simulink model "Vision"  (R2015a)
settings: Solver=ode45  SolverMode=SingleTasking  StartTime=0.0  StopTime=inf  RelTol=1e-3
undefined symbols (not defined in the file or in its folder): gray, none, strel, videoinput
libraries: simulink x12, visiontextngfix x6, visionanalysis x6, visionmorphops x4, visionstatistics x2, visionsinks x2, imaqlib x1
settings Model: CovMetricSettings=dwe  CovHtmlReporting=off  covSaveCumulativeToWorkspaceVar=off  CovSaveSingleToWorkspaceVar=off  CovExternalEMLEnable=on  Creator=Nauj_epilef  LastModifiedBy=Antonio
settings DataIOCC: LimitDataPoints=off  SaveFormat=Dataset
settings DebuggingCC: SFUnexpectedBacktrackingDiag=error  SFNoUnconditionalDefaultTransitionDiag=error
settings HardwareCC: ProdBitPerPointer=64  ProdLargestAtomicFloat=Float  ProdIntDivRoundTo=Zero  ProdEndianess=LittleEndian  ProdHWDeviceType=Specified
settings ModelReferenceCC: PropagateSignalLabelsOutOfModel=on
settings GRTTargetCC: TargetLangStandard=C99 (ISO)  GeneratePreprocessorConditionals=Use local settings

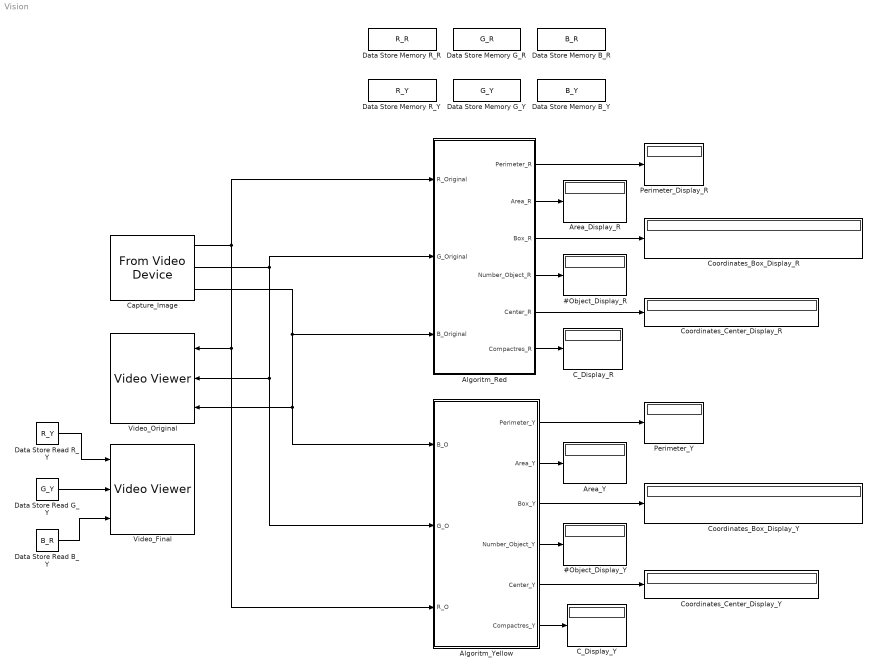
== system Vision ==
  #Object_Display_R : Display
  #Object_Display_Y : Display
  Algoritm_Red : Subsystem
  Algoritm_Yellow : Subsystem
  Area_Display_R : Display
  Area_Y : Display
  C_Display_R : Display
  "C_Display_Y " : Display
  Capture_Image : imaqlib/From Video Device  DeviceMenu=(none)  Device=winvideo 1 (Logitech HD Webcam C525)  ObjConstructor=videoinput('winvideo', 1)  VideoFormatMenu=(none)  VideoFormat=RGB24_640x480  VideoSource=input1  ROIPosition=[184 115 146 417]  EnableHWTrigger=off  TriggerConfiguration=none/none  SampleTime=1/10  OutputPortsMode=Separate color signals  DataType=single  CanDoHWTrigger=no  ReturnedColorSpace=rgb  BlockHandle=645.0004  ROIWidth=417  ROIHeight=146  ROIColumn=115  ROIRow=184  EngXMLPath=C:\Program Files\MATLAB\R2017a\toolbox\imaq\imaq\private  DevXMLPath=C:\ProgramData\MATLAB\SupportPackages\R2017a\toolbox\imaq\supportpackages\genericvideo\adaptor\win64  EngLibPath=C:\Program Files\MATLAB\R2017a\toolbox\imaq\imaqblks\imaqmex\win64  ColorSpace=rgb  BayerSensorAlignment=grbg
  Coordinates_Box_Display_R : Display
  Coordinates_Box_Display_Y : Display
  Coordinates_Center_Display_R : Display
  Coordinates_Center_Display_Y : Display
  Data Store Memory B_R : DataStoreMemory  DataStoreName=B_R  ReadBeforeWriteMsg=warning  WriteAfterWriteMsg=warning  WriteAfterReadMsg=warning  ShowAdditionalParam=off
  Data Store Memory B_Y : DataStoreMemory  DataStoreName=B_Y  ReadBeforeWriteMsg=warning  WriteAfterWriteMsg=warning  WriteAfterReadMsg=warning  ShowAdditionalParam=off
  Data Store Memory G_R : DataStoreMemory  DataStoreName=G_R  ReadBeforeWriteMsg=warning  WriteAfterWriteMsg=warning  WriteAfterReadMsg=warning  ShowAdditionalParam=off
  Data Store Memory G_Y : DataStoreMemory  DataStoreName=G_Y  ReadBeforeWriteMsg=warning  WriteAfterWriteMsg=warning  WriteAfterReadMsg=warning  ShowAdditionalParam=off
  Data Store Memory R_R : DataStoreMemory  DataStoreName=R_R  ReadBeforeWriteMsg=warning  WriteAfterWriteMsg=warning  WriteAfterReadMsg=warning  ShowAdditionalParam=off
  Data Store Memory R_Y : DataStoreMemory  DataStoreName=R_Y  ReadBeforeWriteMsg=warning  WriteAfterWriteMsg=warning  WriteAfterReadMsg=warning  ShowAdditionalParam=off
  "Data Store Read B_Y " : DataStoreRead  DataStoreName=B_R
  Data Store Read G_Y : DataStoreRead  DataStoreName=G_Y
  "Data Store Read R_Y " : DataStoreRead  DataStoreName=R_Y
  Perimeter_Display_R : Display
  Perimeter_Y : Display
  Video_Final : visionsinks/Video Viewer  inputType=Obsolete7b  useColorMap=off  colormapValue=gray(256)  specRange=off  minInputVal=0  maxInputVal=255  FigPos=[1 858 1440 758]  AxisZoom=on  trueSizedOnce=off  OpenAtMdlStart=off  imagePorts=separate color signals
  Video_Original : visionsinks/Video Viewer  inputType=Obsolete7b  useColorMap=off  colormapValue=gray(256)  specRange=off  minInputVal=0  maxInputVal=255  FigPos=[1 898 1440 798]  AxisZoom=on  trueSizedOnce=off  OpenAtMdlStart=off  imagePorts=separate color signals
  wires:
  Capture_Image/1 -> Algoritm_Yellow/3(R_O), Video_Original/1, Algoritm_Red/1(R_Original)
  Capture_Image/3 -> Algoritm_Yellow/1(B_O), Video_Original/3, Algoritm_Red/3(B_Original)
  Capture_Image/2 -> Algoritm_Yellow/2(G_O), Video_Original/2, Algoritm_Red/2(G_Original)
  Algoritm_Red/1("Perimeter_R ") -> Perimeter_Display_R/1
  Algoritm_Red/2(Area_R) -> Area_Display_R/1
  Algoritm_Red/3(Box_R) -> Coordinates_Box_Display_R/1
  Algoritm_Red/4(Number_Object_R) -> #Object_Display_R/1
  Algoritm_Red/5(Center_R) -> Coordinates_Center_Display_R/1
  Algoritm_Red/6(Compactres_R) -> C_Display_R/1
  Algoritm_Yellow/1("Perimeter_Y ") -> Perimeter_Y/1
  Algoritm_Yellow/2(Area_Y) -> Area_Y/1
  "Data Store Read R_Y "/1 -> Video_Final/1
  Data Store Read G_Y/1 -> Video_Final/2
  "Data Store Read B_Y "/1 -> Video_Final/3
  Algoritm_Yellow/6(Compactres_Y) -> "C_Display_Y "/1
  Algoritm_Yellow/3(Box_Y) -> Coordinates_Box_Display_Y/1
  Algoritm_Yellow/4(Number_Object_Y) -> #Object_Display_Y/1
  Algoritm_Yellow/5(Center_Y) -> Coordinates_Center_Display_Y/1

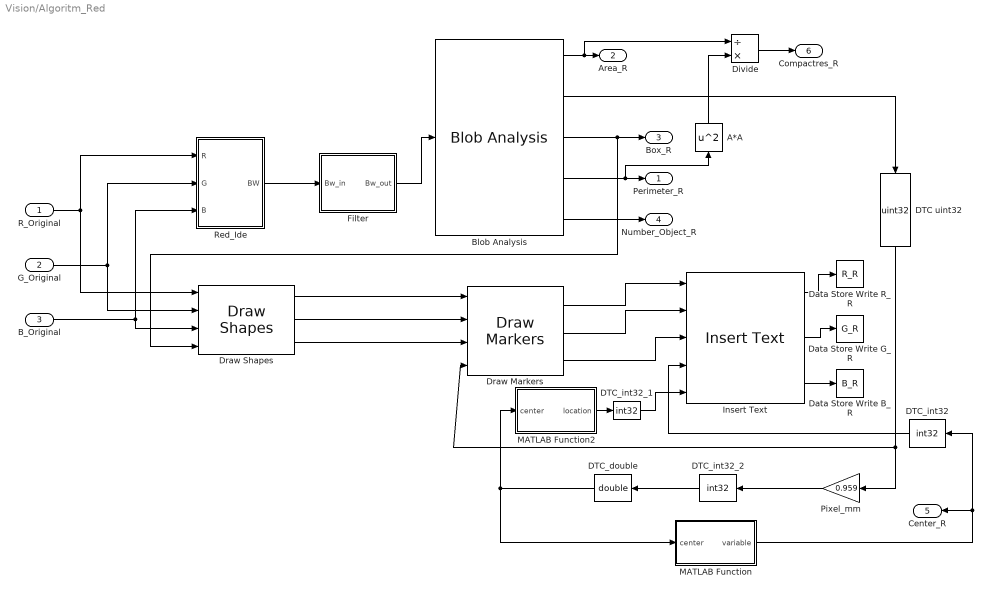
== system Vision/Algoritm_Red ==
  R_Original : Inport
  G_Original : Inport  Port=2
  B_Original : Inport  Port=3
  A*A : Math  Operator=square  SaturateOnIntegerOverflow=on
  Blob Analysis : visionstatistics/Blob Analysis  Tag=vipblks_row_conv  area=on  centroid=on  bBox=on  majorAxis=off  minorAxis=off  angle=off  eccentricity=off  equivDiameterSq=off  extent=off  perimeter=on  maxBlobs=2  warnIfNumBlobsExceeded=on  isCount=on  useMinArea=on  minArea=700  useMaxArea=off  maxArea=intmax('uint32')  excludeBorderBlob=on  outDT=double  isOutVarDim=off  isFill=on  fillValues=-1  conn=8  isLabel=off  outputMode=Binary point scaling  outputWordLength=32  outputFracLength=16  firstCoeffMode=Binary point scaling  firstCoeffWordLength=16  firstCoeffFracLength=14  secondCoeffMode=Binary point scaling  secondCoeffWordLength=32  secondCoeffFracLength=16  accumMode=Binary point scaling  accumWordLength=32  accumFracLength=0  prodOutputMode=Binary point scaling  prodOutputWordLength=32  prodOutputFracLength=16  roundingMode=Floor  overflowMode=off
  DTC uint32 : DataTypeConversion  OutDataTypeStr=uint32
  DTC_double : DataTypeConversion  OutDataTypeStr=double
  DTC_int32 : DataTypeConversion  OutDataTypeStr=int32
  DTC_int32_1 : DataTypeConversion  OutDataTypeStr=int32
  DTC_int32_2 : DataTypeConversion  OutDataTypeStr=int32
  Data Store Write B_R : DataStoreWrite  DataStoreName=B_R
  Data Store Write G_R : DataStoreWrite  DataStoreName=G_R
  Data Store Write R_R : DataStoreWrite  DataStoreName=R_R
  Divide : Product  Inputs=/*
  Draw Markers : visiontextngfix/Draw Markers  shape=Plus  size=8  fill=off  fillClrSource=Specify via dialog  display=User-specified value  intensity=200  color=[0 0 1]  opacity=0.6  viewport=Entire image  antialiasing=off  inType=Obsolete  imagePorts=Separate color signals  prodOutputMode=Binary point scaling  prodOutputWordLength=32  prodOutputFracLength=14  memoryMode=Specify word length  memoryWordLength=16  memoryFracLength=15  roundingMode=Floor  overflowMode=off
  Draw Shapes : visiontextngfix/Draw Shapes  shape=Rectangles  fill=off  lineWidth=1  fillClrSource=Specify via dialog  display=User-specified value  intensity=200  color=[0 0 255]  opacity=0.5  viewport=Entire image  antialiasing=off  inType=Obsolete  imagePorts=Separate color signals  prodOutputMode=Binary point scaling  prodOutputWordLength=32  prodOutputFracLength=14  memoryMode=Specify word length  memoryWordLength=16  memoryFracLength=14  roundingMode=Floor  overflowMode=off
  Filter : Subsystem
  Insert Text : visiontextngfix/Insert Text  inputType=Obsolete  theText='[%i;%i]'  getTextLocFrom=Input port  textLoc=[1 1]  getTextColorFrom=Specify via dialog  textColor=[0 0 0]  getTextIntensityFrom=Specify via dialog  textIntensity=0  getTextOpacityFrom=Specify via dialog  textOpacity=1  dummyVar2=0  dummyVar3=0  dummyVar4=0  imagePorts=Separate color signals  isInputTransposed=off  fontFace=Calibri  dummyVar1=0  blockFontSize=20  antiAliased=on
  MATLAB Function : MATLAB Function  TreatAsAtomicUnit=on
      settings: PermitHierarchicalResolution=ParametersOnly
  MATLAB Function2 : MATLAB Function  TreatAsAtomicUnit=on
      settings: PermitHierarchicalResolution=ParametersOnly
  Pixel_mm : Gain  Gain=0.959
  Red_Ide : Subsystem
  "Perimeter_R " : Outport
  Area_R : Outport  Port=2
  Box_R : Outport  Port=3
  Number_Object_R : Outport  Port=4
  Center_R : Outport  Port=5
  Compactres_R : Outport  Port=6
  wires:
  B_Original/1 -> Draw Shapes/3, Red_Ide/3(B)
  G_Original/1 -> Red_Ide/2(G), Draw Shapes/2
  R_Original/1 -> Draw Shapes/1, Red_Ide/1(R)
  Blob Analysis/5 -> Number_Object_R/1
  Insert Text/1 -> Data Store Write R_R/1
  MATLAB Function/1(variable) -> DTC_int32/1, Center_R/1
  Insert Text/3 -> Data Store Write B_R/1
  Draw Shapes/3 -> Draw Markers/3
  Draw Markers/3 -> Insert Text/3
  Draw Shapes/2 -> Draw Markers/2
  DTC_double/1 -> MATLAB Function/1(center), MATLAB Function2/1(center)
  Blob Analysis/2 -> DTC uint32/1
  Blob Analysis/3 -> Draw Shapes/4, Box_R/1
  Draw Markers/1 -> Insert Text/1
  Red_Ide/1(BW) -> Filter/1(Bw_in)
  DTC_int32_2/1 -> DTC_double/1
  Pixel_mm/1 -> DTC_int32_2/1
  DTC uint32/1 -> Draw Markers/4, Pixel_mm/1
  Draw Shapes/1 -> Draw Markers/1
  Insert Text/2 -> Data Store Write G_R/1
  Filter/1(Bw_out) -> Blob Analysis/1
  Draw Markers/2 -> Insert Text/2
  DTC_int32/1 -> Insert Text/4
  MATLAB Function2/1(location) -> DTC_int32_1/1
  DTC_int32_1/1 -> Insert Text/5
  Blob Analysis/4 -> A*A/1, "Perimeter_R "/1
  Blob Analysis/1 -> Divide/1, Area_R/1
  Divide/1 -> Compactres_R/1
  A*A/1 -> Divide/2

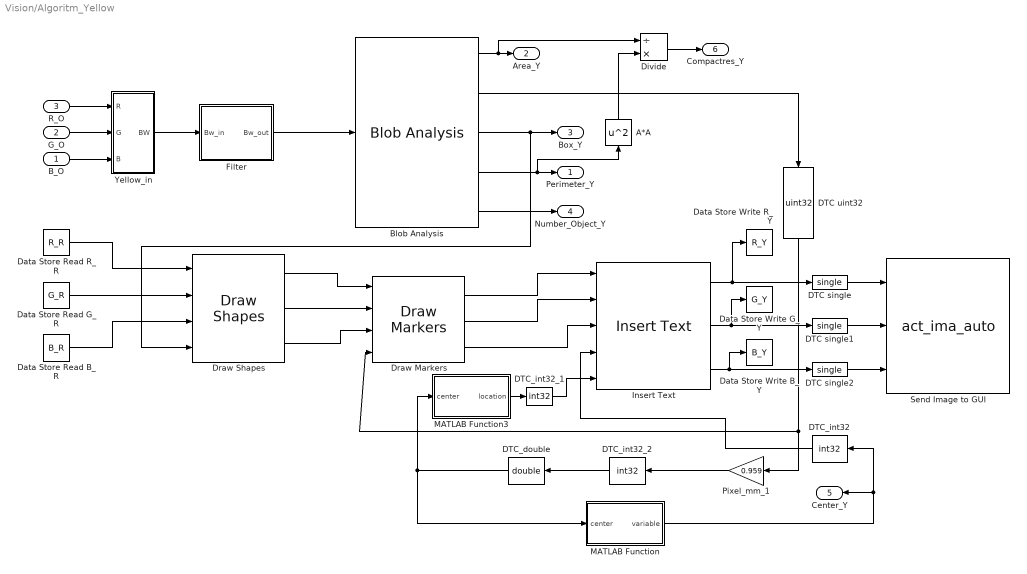
== system Vision/Algoritm_Yellow ==
  B_O : Inport
  G_O : Inport  Port=2
  R_O : Inport  Port=3
  A*A : Math  Operator=square  SaturateOnIntegerOverflow=on
  Blob Analysis : visionstatistics/Blob Analysis  Tag=vipblks_row_conv  area=on  centroid=on  bBox=on  majorAxis=off  minorAxis=off  angle=off  eccentricity=off  equivDiameterSq=off  extent=off  perimeter=on  maxBlobs=2  warnIfNumBlobsExceeded=on  isCount=on  useMinArea=on  minArea=700  useMaxArea=off  maxArea=intmax('uint32')  excludeBorderBlob=on  outDT=double  isOutVarDim=off  isFill=on  fillValues=-1  conn=8  isLabel=off  outputMode=Binary point scaling  outputWordLength=32  outputFracLength=16  firstCoeffMode=Binary point scaling  firstCoeffWordLength=16  firstCoeffFracLength=14  secondCoeffMode=Binary point scaling  secondCoeffWordLength=32  secondCoeffFracLength=16  accumMode=Binary point scaling  accumWordLength=32  accumFracLength=0  prodOutputMode=Binary point scaling  prodOutputWordLength=32  prodOutputFracLength=16  roundingMode=Floor  overflowMode=off
  DTC single : DataTypeConversion  OutDataTypeStr=single
  DTC single1 : DataTypeConversion  OutDataTypeStr=single
  DTC single2 : DataTypeConversion  OutDataTypeStr=single
  DTC uint32 : DataTypeConversion  OutDataTypeStr=uint32
  DTC_double : DataTypeConversion  OutDataTypeStr=double
  DTC_int32 : DataTypeConversion  OutDataTypeStr=int32
  DTC_int32_1 : DataTypeConversion  OutDataTypeStr=int32
  DTC_int32_2 : DataTypeConversion  OutDataTypeStr=int32
  "Data Store Read B_R " : DataStoreRead  DataStoreName=B_R
  Data Store Read G_R : DataStoreRead  DataStoreName=G_R
  Data Store Read R_R : DataStoreRead  DataStoreName=R_R
  Data Store Write B_Y : DataStoreWrite  DataStoreName=B_Y
  Data Store Write G_Y : DataStoreWrite  DataStoreName=G_Y
  Data Store Write R_Y : DataStoreWrite  DataStoreName=R_Y
  Divide : Product  Inputs=/*
  Draw Markers : visiontextngfix/Draw Markers  shape=Plus  size=8  fill=off  fillClrSource=Specify via dialog  display=User-specified value  intensity=200  color=[0 0 1]  opacity=0.6  viewport=Entire image  antialiasing=off  inType=Obsolete  imagePorts=Separate color signals  prodOutputMode=Binary point scaling  prodOutputWordLength=32  prodOutputFracLength=14  memoryMode=Specify word length  memoryWordLength=16  memoryFracLength=15  roundingMode=Floor  overflowMode=off
  Draw Shapes : visiontextngfix/Draw Shapes  shape=Rectangles  fill=off  lineWidth=1  fillClrSource=Specify via dialog  display=User-specified value  intensity=200  color=[0 0 255]  opacity=0.5  viewport=Entire image  antialiasing=off  inType=Obsolete  imagePorts=Separate color signals  prodOutputMode=Binary point scaling  prodOutputWordLength=32  prodOutputFracLength=14  memoryMode=Specify word length  memoryWordLength=16  memoryFracLength=14  roundingMode=Floor  overflowMode=off
  Filter : Subsystem
  Insert Text : visiontextngfix/Insert Text  inputType=Obsolete  theText='[%i;%i]'  getTextLocFrom=Input port  textLoc=[1 1]  getTextColorFrom=Specify via dialog  textColor=[0 0 0]  getTextIntensityFrom=Specify via dialog  textIntensity=0  getTextOpacityFrom=Specify via dialog  textOpacity=1  dummyVar2=0  dummyVar3=0  dummyVar4=0  imagePorts=Separate color signals  isInputTransposed=off  fontFace=Calibri  dummyVar1=0  blockFontSize=20  antiAliased=on
  MATLAB Function : MATLAB Function  TreatAsAtomicUnit=on
      settings: PermitHierarchicalResolution=ParametersOnly
  MATLAB Function3 : MATLAB Function  TreatAsAtomicUnit=on
      settings: PermitHierarchicalResolution=ParametersOnly
  Pixel_mm_1 : Gain  Gain=0.959
  Send Image to GUI : M-S-Function  FunctionName=act_ima_auto
  Yellow_in : Subsystem
  "Perimeter_Y " : Outport
  Area_Y : Outport  Port=2
  Box_Y : Outport  Port=3
  Number_Object_Y : Outport  Port=4
  Center_Y : Outport  Port=5
  Compactres_Y : Outport  Port=6
  wires:
  Yellow_in/1(BW) -> Filter/1(Bw_in)
  B_O/1 -> Yellow_in/3(B)
  G_O/1 -> Yellow_in/2(G)
  R_O/1 -> Yellow_in/1(R)
  Draw Shapes/2 -> Draw Markers/2
  DTC_int32_2/1 -> DTC_double/1
  Blob Analysis/5 -> Number_Object_Y/1
  DTC uint32/1 -> Draw Markers/4, Pixel_mm_1/1
  Draw Markers/1 -> Insert Text/1
  MATLAB Function3/1(location) -> DTC_int32_1/1
  MATLAB Function/1(variable) -> DTC_int32/1, Center_Y/1
  DTC_double/1 -> MATLAB Function/1(center), MATLAB Function3/1(center)
  DTC_int32_1/1 -> Insert Text/5
  Pixel_mm_1/1 -> DTC_int32_2/1
  Blob Analysis/4 -> A*A/1, "Perimeter_Y "/1
  Draw Shapes/1 -> Draw Markers/1
  Draw Markers/3 -> Insert Text/3
  DTC_int32/1 -> Insert Text/4
  Draw Markers/2 -> Insert Text/2
  Blob Analysis/1 -> Divide/1, Area_Y/1
  Insert Text/1 -> Data Store Write R_Y/1, DTC single/1
  Divide/1 -> Compactres_Y/1
  Insert Text/2 -> Data Store Write G_Y/1, DTC single1/1
  Blob Analysis/3 -> Draw Shapes/4, Box_Y/1
  A*A/1 -> Divide/2
  Draw Shapes/3 -> Draw Markers/3
  Insert Text/3 -> Data Store Write B_Y/1, DTC single2/1
  Blob Analysis/2 -> DTC uint32/1
  Filter/1(Bw_out) -> Blob Analysis/1
  Data Store Read R_R/1 -> Draw Shapes/1
  Data Store Read G_R/1 -> Draw Shapes/2
  "Data Store Read B_R "/1 -> Draw Shapes/3
  DTC single2/1 -> Send Image to GUI/3
  DTC single1/1 -> Send Image to GUI/2
  DTC single/1 -> Send Image to GUI/1

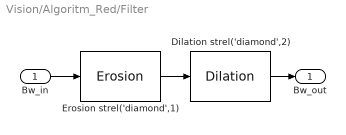
== system Vision/Algoritm_Red/Filter ==
  Bw_in : Inport
  Dilation strel('diamond',2) : visionmorphops/Dilation  nhoodsrc=Specify via dialog  strel=strel('diamond',2)
  Erosion strel('diamond',1) : visionmorphops/Erosion  nhoodsrc=Specify via dialog  strel=strel('diamond',1)
  Bw_out : Outport
  wires:
  Erosion strel('diamond',1)/1 -> Dilation strel('diamond',2)/1
  Bw_in/1 -> Erosion strel('diamond',1)/1
  Dilation strel('diamond',2)/1 -> Bw_out/1

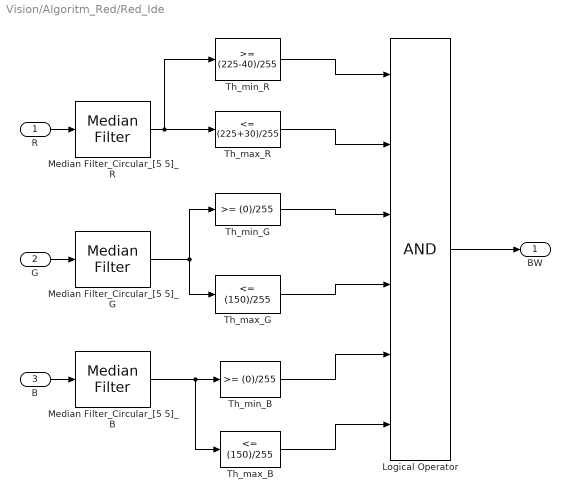
== system Vision/Algoritm_Red/Red_Ide ==
  R : Inport
  G : Inport  Port=2
  B : Inport  Port=3
  Logical Operator : Logic  Inputs=6  AllPortsSameDT=off  OutDataTypeStr=boolean
  Median Filter_Circular_[5 5]_B : visionanalysis/Median Filter  nghbood=[5 5]  outSize=Same as input port I  padType=Circular  padSrc=Specify via dialog  padVal=0  roundingMode=Floor  overflowMode=off
  Median Filter_Circular_[5 5]_G : visionanalysis/Median Filter  nghbood=[5 5]  outSize=Same as input port I  padType=Circular  padSrc=Specify via dialog  padVal=0  roundingMode=Floor  overflowMode=off
  Median Filter_Circular_[5 5]_R : visionanalysis/Median Filter  nghbood=[5 5]  outSize=Same as input port I  padType=Circular  padSrc=Specify via dialog  padVal=0  roundingMode=Floor  overflowMode=off
  Th_max_B : simulink/Logic and Bit Operations/Compare To Constant  relop=<=  const=(150)/255  OutDataTypeStr=boolean
  Th_max_G : simulink/Logic and Bit Operations/Compare To Constant  relop=<=  const=(150)/255  OutDataTypeStr=boolean
  "Th_max_R " : simulink/Logic and Bit Operations/Compare To Constant  relop=<=  const=(225+30)/255  OutDataTypeStr=boolean
  Th_min_B : simulink/Logic and Bit Operations/Compare To Constant  relop=>=  const=(0)/255  OutDataTypeStr=boolean
  Th_min_G : simulink/Logic and Bit Operations/Compare To Constant  relop=>=  const=(0)/255  OutDataTypeStr=boolean
  Th_min_R : simulink/Logic and Bit Operations/Compare To Constant  relop=>=  const=(225-40)/255  OutDataTypeStr=boolean
  BW : Outport
  wires:
  "Th_max_R "/1 -> Logical Operator/2
  Logical Operator/1 -> BW/1
  Th_min_B/1 -> Logical Operator/5
  Th_max_G/1 -> Logical Operator/4
  Th_min_R/1 -> Logical Operator/1
  Th_min_G/1 -> Logical Operator/3
  Th_max_B/1 -> Logical Operator/6
  R/1 -> Median Filter_Circular_[5 5]_R/1
  G/1 -> Median Filter_Circular_[5 5]_G/1
  B/1 -> Median Filter_Circular_[5 5]_B/1
  Median Filter_Circular_[5 5]_R/1 -> "Th_max_R "/1, Th_min_R/1
  Median Filter_Circular_[5 5]_G/1 -> Th_max_G/1, Th_min_G/1
  Median Filter_Circular_[5 5]_B/1 -> Th_max_B/1, Th_min_B/1

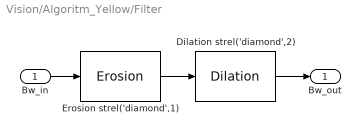
== system Vision/Algoritm_Yellow/Filter ==
  Bw_in : Inport
  Dilation strel('diamond',2) : visionmorphops/Dilation  nhoodsrc=Specify via dialog  strel=strel('diamond',2)
  Erosion strel('diamond',1) : visionmorphops/Erosion  nhoodsrc=Specify via dialog  strel=strel('diamond',1)
  Bw_out : Outport
  wires:
  Erosion strel('diamond',1)/1 -> Dilation strel('diamond',2)/1
  Bw_in/1 -> Erosion strel('diamond',1)/1
  Dilation strel('diamond',2)/1 -> Bw_out/1

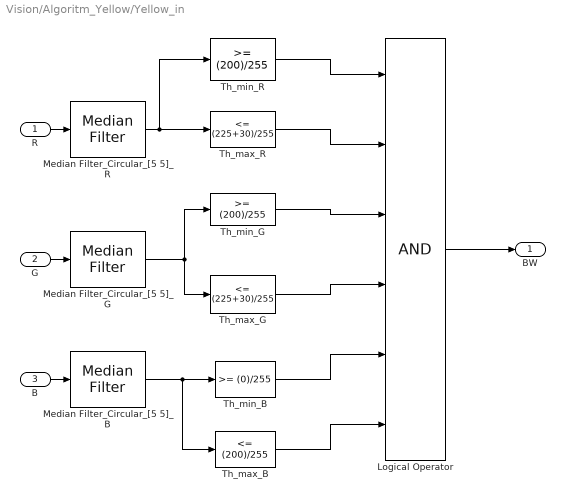
== system Vision/Algoritm_Yellow/Yellow_in ==
  R : Inport
  G : Inport  Port=2
  B : Inport  Port=3
  Logical Operator : Logic  Inputs=6  AllPortsSameDT=off  OutDataTypeStr=boolean
  Median Filter_Circular_[5 5]_B : visionanalysis/Median Filter  nghbood=[5 5]  outSize=Same as input port I  padType=Circular  padSrc=Specify via dialog  padVal=0  roundingMode=Floor  overflowMode=off
  Median Filter_Circular_[5 5]_G : visionanalysis/Median Filter  nghbood=[5 5]  outSize=Same as input port I  padType=Circular  padSrc=Specify via dialog  padVal=0  roundingMode=Floor  overflowMode=off
  Median Filter_Circular_[5 5]_R : visionanalysis/Median Filter  nghbood=[5 5]  outSize=Same as input port I  padType=Circular  padSrc=Specify via dialog  padVal=0  roundingMode=Floor  overflowMode=off
  Th_max_B : simulink/Logic and Bit Operations/Compare To Constant  relop=<=  const=(200)/255  OutDataTypeStr=boolean
  Th_max_G : simulink/Logic and Bit Operations/Compare To Constant  relop=<=  const=(225+30)/255  OutDataTypeStr=boolean
  Th_max_R : simulink/Logic and Bit Operations/Compare To Constant  relop=<=  const=(225+30)/255  OutDataTypeStr=boolean
  Th_min_B : simulink/Logic and Bit Operations/Compare To Constant  relop=>=  const=(0)/255  OutDataTypeStr=boolean
  "Th_min_G " : simulink/Logic and Bit Operations/Compare To Constant  relop=>=  const=(200)/255  OutDataTypeStr=boolean
  "Th_min_R " : simulink/Logic and Bit Operations/Compare To Constant  relop=>=  const=(200)/255  OutDataTypeStr=boolean
  BW : Outport
  wires:
  Th_max_R/1 -> Logical Operator/2
  Logical Operator/1 -> BW/1
  Th_min_B/1 -> Logical Operator/5
  Th_max_G/1 -> Logical Operator/4
  "Th_min_R "/1 -> Logical Operator/1
  "Th_min_G "/1 -> Logical Operator/3
  Th_max_B/1 -> Logical Operator/6
  G/1 -> Median Filter_Circular_[5 5]_G/1
  R/1 -> Median Filter_Circular_[5 5]_R/1
  B/1 -> Median Filter_Circular_[5 5]_B/1
  Median Filter_Circular_[5 5]_R/1 -> "Th_min_R "/1, Th_max_R/1
  Median Filter_Circular_[5 5]_G/1 -> Th_max_G/1, "Th_min_G "/1
  Median Filter_Circular_[5 5]_B/1 -> Th_max_B/1, Th_min_B/1

== matlab function Vision/Algoritm_Red/MATLAB Function ==
  data: center input; variable output
function variable = transpuesta(center)
%High camara
h_camara=700;
%High object
h_objeto=55;
%Split Matrix
c1=center(:,1); %%x
c2=center(:,2); %%y
%Distance center WorkSpace
d=[200;200];
d1=typecast(d,'double');
%Correction x position 
c12=-c1+d1;
x_error=(h_objeto/h_camara)*c12;
x_objeto=c12-x_error;
%Correction y position
%Split vector
c21=c2(1,:);
c22=c2(2,:);
y_error1=(h_objeto/h_camara)*c21*(1/2);
y_error2=(h_objeto/h_camara)*c22*(1/2);
%Condition of correction object_1
if(c21>70)
  y_objeto1=c21-y_error1;
else
  y_objeto1=c21+y_error1;   
end
%Condition of correction object_2
if(c22>70)
  y_objeto2=c22-y_error2;
else
  y_objeto2=c22+y_error2;   
end
y_objeto=[y_objeto1;y_objeto2];
%Ouput x_object  and y_object
n=[x_objeto,y_objeto];
%Transpose
v=n';
variable = [v];

== matlab function Vision/Algoritm_Red/MATLAB Function2 ==
  data: center input; location output
function location = transpuesta(center)
%Split Matrix
c1=center(:,1); %%x
c2=center(:,2);  %%y

dx=[25;25];
dy=35;
%Convert dx and dy to double
dx1=typecast(dx,'double');
dy1=typecast(dy,'double');
%Correction x
x=c1-dx1;
%Correction y
c2_1=c2(1,:);
c2_2=c2(2,:);

if (c2_1>=70)
    c2_11=c2_1-dy1;
else 
    c2_11=c2_1+dy1;
end

if (c2_2>=70)
    c2_21=c2_2-dy1;
else 
    c2_21=c2_2+dy1;
end
y=[c2_11;c2_21];
%Ouput x_object  and y_object
n=[x,y];
location = [n];

== matlab function Vision/Algoritm_Yellow/MATLAB Function ==
  data: center input; variable output
function variable = transpuesta(center)
%High camara
h_camara=700;
%High object
h_objeto=55;
%Split Matrix
c1=center(:,1); %%x
c2=center(:,2); %%y
%Distance center WorkSpace
d=[200;200];
d1=typecast(d,'double');
%Correction x position 
c12=-c1+d1;
x_error=(h_objeto/h_camara)*c12;
x_objeto=c12-x_error;
%Correction y position
%Split vector
c21=c2(1,:);
c22=c2(2,:);
y_error1=(h_objeto/h_camara)*c21*(1/2);
y_error2=(h_objeto/h_camara)*c22*(1/2);
%Condition of correction object_1
if(c21>70)
  y_objeto1=c21-y_error1;
else
  y_objeto1=c21+y_error1;   
end
%Condition of correction object_2
if(c22>70)
  y_objeto2=c22-y_error2;
else
  y_objeto2=c22+y_error2;   
end
y_objeto=[y_objeto1;y_objeto2];
%Ouput x_object  and y_object
n=[x_objeto,y_objeto];
%Transpose
v=n';
variable = [v];

== matlab function Vision/Algoritm_Yellow/MATLAB Function3 ==
  data: center input; location output
function location = transpuesta(center)
%Split Matrix
c1=center(:,1); %%x
c2=center(:,2);  %%y

dx=[25;25];
dy=35;
%Convert dx and dy to double
dx1=typecast(dx,'double');
dy1=typecast(dy,'double');
%Correction x
x=c1-dx1;
%Correction y
c2_1=c2(1,:);
c2_2=c2(2,:);

if (c2_1>=70)
    c2_11=c2_1-dy1;
else 
    c2_11=c2_1+dy1;
end

if (c2_2>=70)
    c2_21=c2_2-dy1;
else 
    c2_21=c2_2+dy1;
end
y=[c2_11;c2_21];
%Ouput x_object  and y_object
n=[x,y];
location = [n];
